simulink model "Ex9_6model"  (R2013a)
settings: Solver=ode45  StartTime=0.0  StopTime=2  RelTol=1e-3
settings Model: Creator=John  LastModifiedBy=John
settings DataIOCC: SignalLoggingSaveFormat=ModelDataLogs
settings OptimizationCC: ExpressionDepthLimit=2147483647
settings DebuggingCC: FcnCallInpInsideContextMsg=UseLocalSettings  StrictBusMsg=Warning
settings GRTTargetCC: CombineOutputUpdateFcns=off  GRTInterface=on

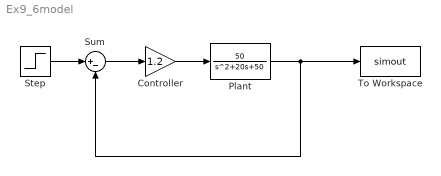
== system Ex9_6model ==
  Controller : Gain  Gain=1.2
  Plant : TransferFcn  Numerator=[50]  Denominator=[1 20 50]
  Step : Step  Time=0  SampleTime=0
  Sum : Sum  Inputs=|+-
  To Workspace : ToWorkspace  VariableName=simout  SampleTime=-1
  wires:
  Plant/1 -> To Workspace/1, Sum/2
  Sum/1 -> Controller/1
  Step/1 -> Sum/1
  Controller/1 -> Plant/1
